simulink model "tralala"  (R2019a)
settings: Solver=FixedStepAuto  StartTime=0.0  StopTime=100  FixedStep=10  RelTol=1e-3
values from neighbouring files (symbols this model uses):
  e0 = 1    [skrypt_01.m]
  e1 = 1    [skrypt_01.m]
  eks_1 = 1    [skrypt_01.m]
  eks_2 = 1    [skrypt_01.m]
  h = 0.05    [skrypt_01.m]
  k = 1    [skrypt_01.m]
  k_1 = 0.5    [skrypt_01.m]
  k_3 = 0.03445    [skrypt_01.m]
  N = 0.1    [skrypt_01.m]
  r = 1    [skrypt_01.m]
  T = 1    [skrypt_01.m]
libraries: simulink x1
settings Model: Creator=podstawy  LastModifiedBy=wojte
settings DataIOCC: ReturnWorkspaceOutputs=off
settings DebuggingCC: ArithmeticOperatorsInVariantConditions=warning

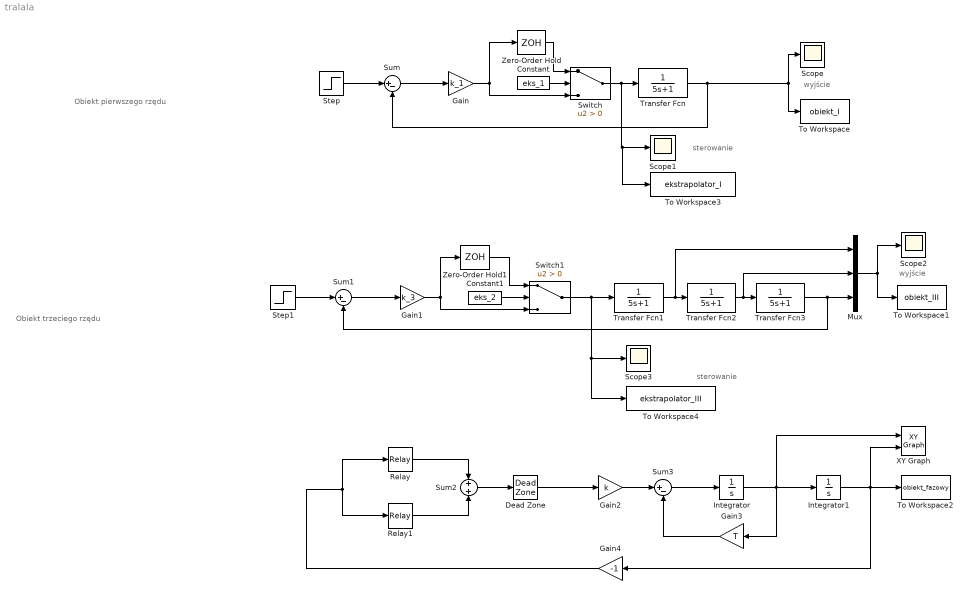
== system tralala ==
  note: sterowanie
  note: wyjście
  note: Obiekt trzeciego rzędu
  note: Obiekt pierwszego rzędu
  note: wyjście
  note: sterowanie
  Constant : Constant  Value=eks_1
  Constant1 : Constant  Value=eks_2
  Dead Zone : DeadZone  LowerValue=-N  UpperValue=N  SaturateOnIntegerOverflow=on
  Gain : Gain  Gain=k_1
  Gain1 : Gain  Gain=k_3
  Gain2 : Gain  Gain=k
  Gain3 : Gain  Gain=T
  Gain4 : Gain  Gain=-1
  Integrator : Integrator  InitialCondition=e1
  Integrator1 : Integrator  InitialCondition=e0
  Mux : Mux  Inputs=3
  Relay : Relay  OnSwitchValue=N+h  OffSwitchValue=N
  Relay1 : Relay  OnSwitchValue=-N  OffSwitchValue=-N-h  OnOutputValue=0  OffOutputValue=-1
  Scope{,1..3} (4 alike) : Scope
  Step : Step  After=r  SampleTime=0
  Step1 : Step  After=r  SampleTime=0
  Sum : Sum  Inputs=|+-
  Sum1 : Sum  Inputs=|+-
  Sum2 : Sum
  Sum3 : Sum  Inputs=|+-
  Switch : Switch  Criteria=u2 > Threshold
  Switch1 : Switch  Criteria=u2 > Threshold
  To Workspace : ToWorkspace  VariableName=obiekt_I  SaveFormat=Timeseries  SampleTime=-1
  To Workspace1 : ToWorkspace  VariableName=obiekt_III  SaveFormat=Timeseries  SampleTime=-1
  To Workspace2 : ToWorkspace  VariableName=obiekt_fazowy  SaveFormat=Timeseries  SampleTime=-1
  To Workspace3 : ToWorkspace  VariableName=ekstrapolator_I  SaveFormat=Timeseries  SampleTime=-1
  To Workspace4 : ToWorkspace  VariableName=ekstrapolator_III  SaveFormat=Timeseries  SampleTime=-1
  Transfer Fcn{,1..3} (4 alike) : TransferFcn  Denominator=[5 1]
  XY Graph : simulink/Sinks/XY Graph  xmin=-1  xmax=1  ymin=-1  ymax=1  st=-1
  Zero-Order Hold : ZeroOrderHold  SampleTime=-1
  Zero-Order Hold1 : ZeroOrderHold  SampleTime=-1
  wires:
  Sum/1 -> Gain/1
  Step/1 -> Sum/1
  Transfer Fcn/1 -> Sum/2, To Workspace/1, Scope/1
  Step1/1 -> Sum1/1
  Sum1/1 -> Gain1/1
  Transfer Fcn1/1 -> Mux/1, Transfer Fcn2/1
  Transfer Fcn2/1 -> Mux/2, Transfer Fcn3/1
  Switch1/1 -> Transfer Fcn1/1, To Workspace4/1, Scope3/1
  Mux/1 -> To Workspace1/1, Scope2/1
  Transfer Fcn3/1 -> Sum1/2, Mux/3
  Gain1/1 -> Switch1/3, Zero-Order Hold1/1
  Zero-Order Hold1/1 -> Switch1/1
  Constant1/1 -> Switch1/2
  Gain/1 -> Switch/3, Zero-Order Hold/1
  Constant/1 -> Switch/2
  Switch/1 -> To Workspace3/1, Scope1/1, Transfer Fcn/1
  Zero-Order Hold/1 -> Switch/1
  Relay/1 -> Sum2/1
  Relay1/1 -> Sum2/2
  Sum2/1 -> Dead Zone/1
  Dead Zone/1 -> Gain2/1
  Gain2/1 -> Sum3/1
  Sum3/1 -> Integrator/1
  Gain3/1 -> Sum3/2
  Integrator/1 -> Integrator1/1, XY Graph/1, Gain3/1
  Integrator1/1 -> Gain4/1, XY Graph/2, To Workspace2/1
  Gain4/1 -> Relay1/1, Relay/1
